simulink model "sl_ctorque2"  (Simulink 7.7)
settings: Solver=ode45  StartTime=0.0  StopTime=10.0  FixedStep=0.01  RelTol=1e-3
PreLoadFcn:
  | puma560
  | p560 = nofriction(p560);
libraries: roblocks x2,  x1
settings Model: Creator=pic  LastModifiedBy=corkep  ExtModeTrigMode=oneshot  ExtModeArmWhenConnect=off
settings DataIOCC: LimitDataPoints=off  ReturnWorkspaceOutputs=on
settings OptimizationCC: BlockReduction=off  BooleanDataType=off  InitFltsAndDblsToZero=on
settings DebuggingCC: SaveWithParameterizedLinksMsg=none  SignalResolutionControl=TryResolveAllWithWarning  SolverPrmCheckMsg=none  MultiTaskDSMMsg=warning  MultiTaskCondExecSysMsg=none  StrictBusMsg=None
settings HardwareCC: TargetUnknown=on
settings RTWCC: IncludeERTFirstTime=on
settings GRTTargetCC: ModelReferenceCompliant=off  CompOptLevelCompliant=off  MatFileLogging=off

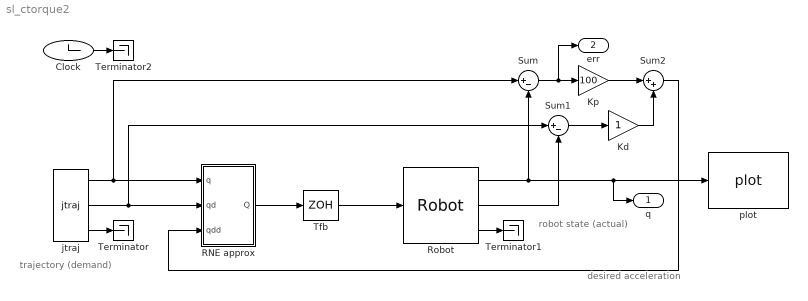
== system sl_ctorque2 ==
  note: trajectory
      | (demand)
  note: robot state
      | (actual)
  note: desired acceleration
  Clock : Clock
      settings: Decimation=10
  Kd : Gain  SaturateOnIntegerOverflow=on  OutDataTypeStr=Inherit: Same as input  ParamDataTypeStr=Inherit: Same as input
  Kp : Gain  Gain=100  SaturateOnIntegerOverflow=on  OutDataTypeStr=Inherit: Same as input  ParamDataTypeStr=Inherit: Same as input
  RNE approx : Subsystem  mask{robot=p560, ts=0.05}
      mask prompts: ts "Sample interval (s)"
  Robot : /Dynamics/Robot  SystemSampleTime=-1  robot=p560.nofriction()  q0=[0 0 0 0 0 0]
  Sum : Sum  Inputs=|+-  SaturateOnIntegerOverflow=on  InputSameDT=on  OutDataTypeStr=Inherit: Same as first input
  Sum1 : Sum  Inputs=|+-  SaturateOnIntegerOverflow=on  InputSameDT=on  OutDataTypeStr=Inherit: Same as first input
  Sum2 : Sum  Inputs=|++  SaturateOnIntegerOverflow=on  InputSameDT=on  OutDataTypeStr=Inherit: Same as first input
  Terminator : Terminator
  Terminator1 : Terminator
  Terminator2 : Terminator
  Tfb : ZeroOrderHold  SampleTime=0.01
  jtraj : roblocks/Trajectory/jtraj  SystemSampleTime=-1  q0=[0 0 0 0 0 0]  qf=[pi/4 pi/2 -pi/2 0 0 0]  tmax=10  ts=0.02
  plot : roblocks/Robot Graphics/plot  SystemSampleTime=-1  robot=p560  fps=25
  q : Outport
  err : Outport  Port=2
  wires:
  Sum/1 -> Kp/1, err/1
  Kp/1 -> Sum2/1
  Robot/1 -> Sum/2, q/1, plot/1
  Robot/2 -> Sum1/2
  Sum2/1 -> RNE approx/3(qdd)
  RNE approx/1(Q) -> Tfb/1
  jtraj/1 -> Sum/1, RNE approx/1(q)
  jtraj/2 -> Sum1/1, RNE approx/2(qd)
  Sum1/1 -> Kd/1
  Kd/1 -> Sum2/2
  jtraj/3 -> Terminator/1
  Robot/3 -> Terminator1/1
  Tfb/1 -> Robot/1
  Clock/1 -> Terminator2/1

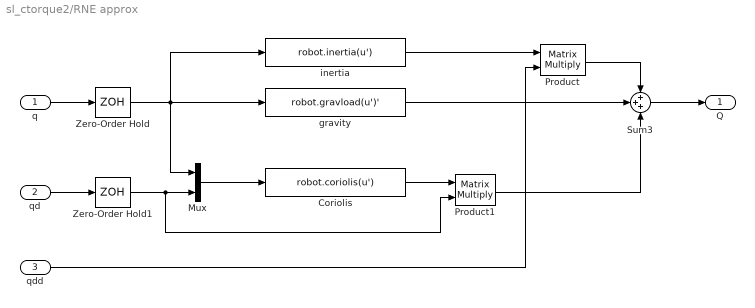
== system sl_ctorque2/RNE approx ==
  q : Inport
  qd : Inport  Port=2
  qdd : Inport  Port=3
  Coriolis : MATLABFcn  MATLABFcn=robot.coriolis(u')  OutputDimensions=[robot.n robot.n]  Output1D=off
  Mux : Mux  Inputs=2
  Product : Product  Multiplication=Matrix(*)  RndMeth=Zero
  Product1 : Product  Multiplication=Matrix(*)  RndMeth=Zero
  Sum3 : Sum  Inputs=+++
  Zero-Order Hold : ZeroOrderHold  SampleTime=ts
  Zero-Order Hold1 : ZeroOrderHold  SampleTime=ts
  gravity : MATLABFcn  MATLABFcn=robot.gravload(u')'  Output1D=off
  inertia : MATLABFcn  MATLABFcn=robot.inertia(u')  OutputDimensions=[robot.n robot.n]  Output1D=off
  Q : Outport
  wires:
  q/1 -> Zero-Order Hold/1
  qd/1 -> Zero-Order Hold1/1
  Zero-Order Hold/1 -> gravity/1, Mux/1, inertia/1
  Zero-Order Hold1/1 -> Mux/2, Product1/2
  inertia/1 -> Product/1
  Mux/1 -> Coriolis/1
  Coriolis/1 -> Product1/1
  Product1/1 -> Sum3/3
  Product/1 -> Sum3/1
  gravity/1 -> Sum3/2
  qdd/1 -> Product/2
  Sum3/1 -> Q/1
